simulink model "TST_ArraySelectors"  (Simulink 7.4)
settings: Solver=FixedStepDiscrete  StartTime=0.0  StopTime=10.0  FixedStep=0.02  RelTol=1e-3
settings Model: Creator=kharthforeign  LastModifiedBy=kharthforeign  BufferReuse=off
settings DataIOCC: SaveOutput=off  SignalLogging=off  SaveTime=off
settings OptimizationCC: BlockReduction=off  ConditionallyExecuteInputs=off  OptimizeBlockIOStorage=off  BufferReuse=off  ExpressionFolding=off  LocalBlockOutputs=off  InitFltsAndDblsToZero=on

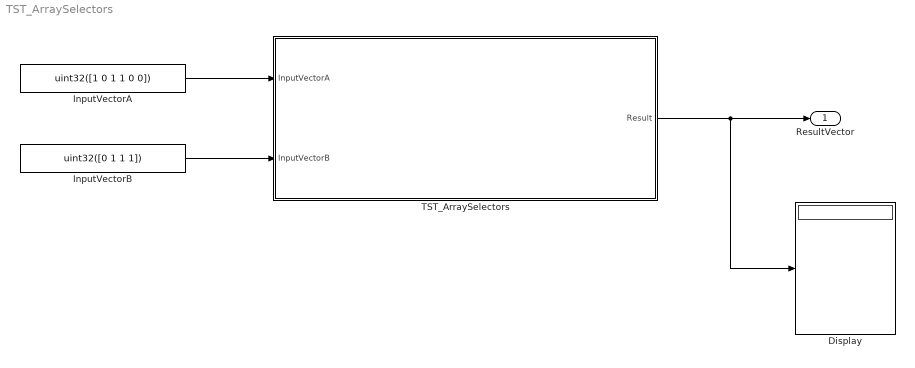
== system TST_ArraySelectors ==
  Display : Display
  InputVectorA : Constant  Value=uint32([1 0 1 1 0 0])  OutDataType=fixdt(1, 16)  OutScaling=2^0
  InputVectorB : Constant  Value=uint32([0 1 1 1])  OutDataType=fixdt(1, 16)  OutScaling=2^0
  TST_ArraySelectors : Subsystem  TreatAsAtomicUnit=on
  ResultVector : Outport  OutDataType=fixdt(1, 16)  OutScaling=2^0
  wires:
  TST_ArraySelectors/1(Result) -> ResultVector/1, Display/1
  InputVectorA/1 -> TST_ArraySelectors/1(InputVectorA)
  InputVectorB/1 -> TST_ArraySelectors/2(InputVectorB)

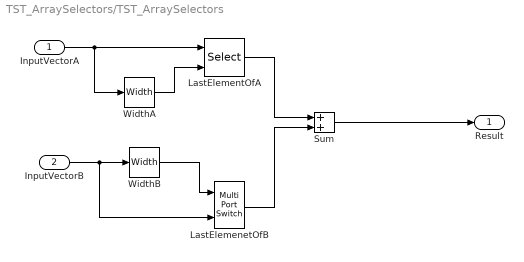
== system TST_ArraySelectors/TST_ArraySelectors ==
  InputVectorA : Inport  OutDataType=fixdt(1, 16)  OutScaling=2^0
  InputVectorB : Inport  Port=2  OutDataType=fixdt(1, 16)  OutScaling=2^0
  LastElemenetOfB : MultiPortSwitch  Inputs=1  OutDataType=fixdt(1, 16)  OutScaling=2^0
  LastElementOfA : Selector  IndexOptions=Index vector (port)  Indices=[1 3]  OutputSizes=1
  Sum : Sum  OutDataType=fixdt(1, 16)  OutScaling=2^0
  WidthA : Width
  WidthB : Width
  Result : Outport  OutDataType=fixdt(1, 16)  OutScaling=2^0
  wires:
  Sum/1 -> Result/1
  InputVectorA/1 -> WidthA/1, LastElementOfA/1
  WidthA/1 -> LastElementOfA/2
  InputVectorB/1 -> WidthB/1, LastElemenetOfB/2
  WidthB/1 -> LastElemenetOfB/1
  LastElementOfA/1 -> Sum/1
  LastElemenetOfB/1 -> Sum/2
